simulink model "np"  (R2024a)
settings: Solver=VariableStepAuto  StartTime=0.0  StopTime=4000  RelTol=1e-3
libraries: aerolibatmos2 x25, simulink x1
(part 2 of 3)

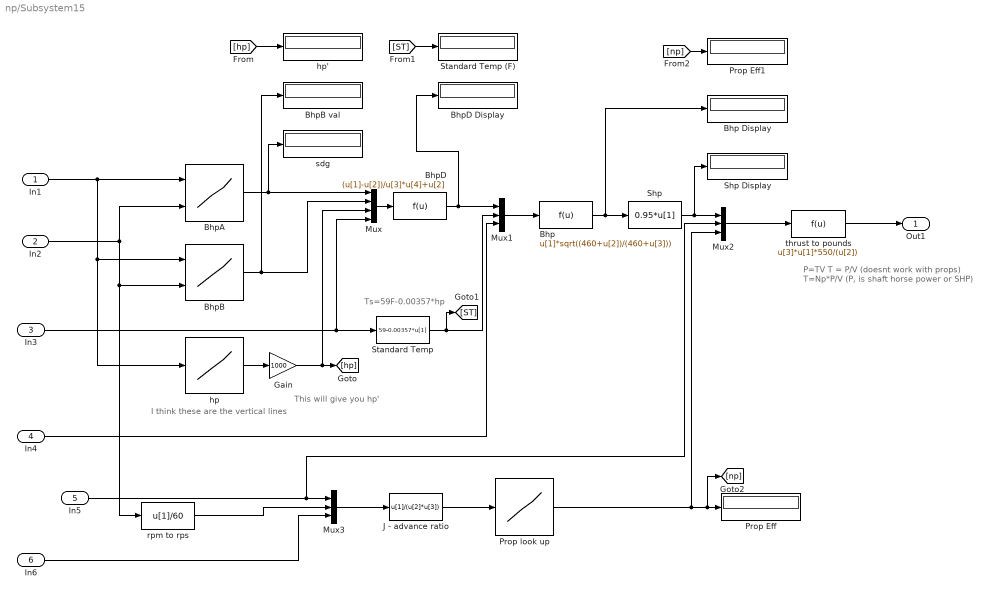
== system np/Subsystem15 ==
  note: This will give you hp'
  note: P=TV
      |
      | T = P/V (doesnt work with props)
      | T=Np*P/V (P, is shaft horse power or SHP)
  note: Ts=59F-0.00357*hp
  note: I think these are the vertical lines
  In1 : Inport
  In2 : Inport  Port=2
  In3 : Inport  Port=3
  In4 : Inport  Port=4
  In5 : Inport  Port=5
  In6 : Inport  Port=6
  Bhp : Fcn  Expr=u[1]*sqrt((460+u[2])/(460+u[3]))
  Bhp Display : Display
  BhpA : Lookup_n-D  BreakpointsForDimension1=[12;14;16;18;20;22;24;26;28]  BreakpointsForDimension2=[2000 2200 2400 2600 2700]  Table=[55 65 68 70 71;69 77 82 84 87;79 87 94 97 100;88 98 105 111 115;98 108 116 123 126;108 119 127 135 140;119 129 138 147 153;127 139 150 160 164;138 149 161 172 177]  InternalRulePriority=Speed  RndMeth=Simplest
      settings: InputPortMap=u0,u1
  BhpB : Lookup_n-D  BreakpointsForDimension1=[17 18 19 20 21 22 23 24 25 26 27 28 29]  BreakpointsForDimension2=[2000 2200 2400 2600 2700]  Table=[60 68 71 81 82;65 74 80 98 90;73 81 86 95 98;80 87 94 103 106;85 95 102 111 116;93 103 110 120 123;100 110 118 126 133;106 115 125 135 141;116 124 135 144 150;120 131 143 152 158;125 137 148 159 165;135 145 157 167 173;142 153 165 176 183]  InternalRulePriority=Speed  RndMeth=Simplest
      settings: InputPortMap=u0,u1
  BhpB val : Display
  BhpD : Fcn  Expr=(u[1]-u[2])/u[3]*u[4]+u[2]
  BhpD Display : Display
  Gain : Gain  Gain=1000
  J - advance ratio : Fcn  Expr=u[1]/(u[2]*u[3])
  Mux : Mux
  Mux1 : Mux  Inputs=3
  Mux2 : Mux  Inputs=3
  Mux3 : Mux  Inputs=3
  Prop Eff : Display
  Prop Eff1 : Display
  Prop look up : Lookup_n-D  NumberOfTableDimensions=1  BreakpointsForDimension1=[0;0.048012249;0.060807878;0.079983697;0.105563205;0.133281193;0.157430152;0.178753263;0.199368443;0.215001671;0.227800237;0.245557257;0.273971426;0.300949171;0.327207235;0.352754431;0.371192944;0.390339388;0.409494645;0.433608354;0.457002383;0.472603298;0.491041811;0.509471512;0.534281402;0.552003172;0.576810125;0.598782418;0.619332973;0.645549913;0.671763915;0.690895672;0.717103799;0.745432781;0.760302266;0.778708467;0.799946391;0.819051711;0.845926644;0.867848999;0.888343743;0.903180915;0.92013013;0.934250559;0.947645432;0.961736487;0.970184657;0.980736057;0.986337817;0.992650444;0.994753675]  Table=[0;0.109900628;0.134509301;0.163123953;0.206809061;0.257361734;0.294163365;0.333794761;0.373442069;0.400753217;0.42674495;0.454008364;0.499012887;0.534367813;0.564206411;0.592677861;0.607477825;0.622261878;0.641195111;0.661400024;0.676088609;0.688186099;0.702986063;0.713636848;0.72829361;0.738960306;0.752234009;0.764188297;0.773408288;0.783884048;0.792976749;0.800845502;0.807172083;0.81206787;0.813116793;0.812703099;0.812225759;0.807646975;0.794594806;0.783037077;0.765978931;0.751814195;0.732069486;0.713771482;0.68719103;0.655062427;0.632742534;0.600693488;0.571521941;0.543717542;0.53398839]  InternalRulePriority=Speed  RndMeth=Simplest
  Shp : Fcn  Expr=0.95*u[1]
  Shp Display : Display
  Standard Temp : Fcn  Expr=59-0.00357*u[1]
  Standard Temp (F) : Display
  hp : Lookup_n-D  NumberOfTableDimensions=1  BreakpointsForDimension1=[12, 14, 16, 18, 20, 22, 24, 26, 28]  Table=[22.5, 19.3, 15.8, 12.8, 10.3, 7.8, 5.5, 3.25, 1.4]  InternalRulePriority=Speed  RndMeth=Simplest
  "hp' " : Display
  rpm to rps : Fcn  Expr=u[1]/60
  sdg : Display
  thrust to pounds : Fcn  Expr=u[3]*u[1]*550/(u[2])
  Out1 : Outport
  wires:
  In6/1 -> Mux3/3
  In4/1 -> Mux1/3
  BhpA/1 -> Mux/1, sdg/1
  BhpD/1 -> Mux1/1, BhpD Display/1
  Mux2/1 -> thrust to pounds/1
  In5/1 -> Mux3/1, Mux2/2
  Bhp/1 -> Shp/1, Bhp Display/1
  thrust to pounds/1 -> Out1/1
  In3/1 -> Standard Temp/1, Mux/4
  Standard Temp/1 -> Mux1/2, [ST]
  BhpB/1 -> Mux/2, BhpB val/1
  Mux1/1 -> Bhp/1
  In2/1 -> rpm to rps/1, BhpB/2, BhpA/2
  In1/1 -> BhpA/1, BhpB/1, hp/1
  Shp/1 -> Mux2/1, Shp Display/1
  [np] -> Prop Eff1/1
  J - advance ratio/1 -> Prop look up/1
  Prop look up/1 -> Mux2/3, Prop Eff/1, [np]
  Mux/1 -> BhpD/1
  rpm to rps/1 -> Mux3/2
  [hp] -> "hp' "/1
  Mux3/1 -> J - advance ratio/1
  [ST] -> Standard Temp (F)/1
  Gain/1 -> Mux/3, [hp]
  hp/1 -> Gain/1

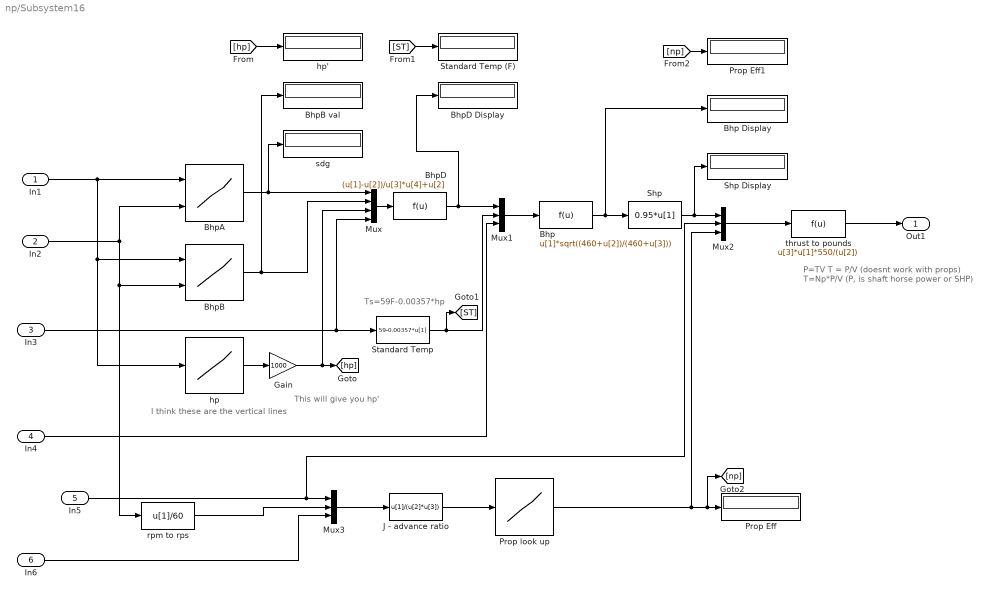
== system np/Subsystem16 ==
  note: This will give you hp'
  note: P=TV
      |
      | T = P/V (doesnt work with props)
      | T=Np*P/V (P, is shaft horse power or SHP)
  note: Ts=59F-0.00357*hp
  note: I think these are the vertical lines
  In1 : Inport
  In2 : Inport  Port=2
  In3 : Inport  Port=3
  In4 : Inport  Port=4
  In5 : Inport  Port=5
  In6 : Inport  Port=6
  Bhp : Fcn  Expr=u[1]*sqrt((460+u[2])/(460+u[3]))
  Bhp Display : Display
  BhpA : Lookup_n-D  BreakpointsForDimension1=[12;14;16;18;20;22;24;26;28]  BreakpointsForDimension2=[2000 2200 2400 2600 2700]  Table=[55 65 68 70 71;69 77 82 84 87;79 87 94 97 100;88 98 105 111 115;98 108 116 123 126;108 119 127 135 140;119 129 138 147 153;127 139 150 160 164;138 149 161 172 177]  InternalRulePriority=Speed  RndMeth=Simplest
      settings: InputPortMap=u0,u1
  BhpB : Lookup_n-D  BreakpointsForDimension1=[17 18 19 20 21 22 23 24 25 26 27 28 29]  BreakpointsForDimension2=[2000 2200 2400 2600 2700]  Table=[60 68 71 81 82;65 74 80 98 90;73 81 86 95 98;80 87 94 103 106;85 95 102 111 116;93 103 110 120 123;100 110 118 126 133;106 115 125 135 141;116 124 135 144 150;120 131 143 152 158;125 137 148 159 165;135 145 157 167 173;142 153 165 176 183]  InternalRulePriority=Speed  RndMeth=Simplest
      settings: InputPortMap=u0,u1
  BhpB val : Display
  BhpD : Fcn  Expr=(u[1]-u[2])/u[3]*u[4]+u[2]
  BhpD Display : Display
  Gain : Gain  Gain=1000
  J - advance ratio : Fcn  Expr=u[1]/(u[2]*u[3])
  Mux : Mux
  Mux1 : Mux  Inputs=3
  Mux2 : Mux  Inputs=3
  Mux3 : Mux  Inputs=3
  Prop Eff : Display
  Prop Eff1 : Display
  Prop look up : Lookup_n-D  NumberOfTableDimensions=1  BreakpointsForDimension1=[0;0.048012249;0.060807878;0.079983697;0.105563205;0.133281193;0.157430152;0.178753263;0.199368443;0.215001671;0.227800237;0.245557257;0.273971426;0.300949171;0.327207235;0.352754431;0.371192944;0.390339388;0.409494645;0.433608354;0.457002383;0.472603298;0.491041811;0.509471512;0.534281402;0.552003172;0.576810125;0.598782418;0.619332973;0.645549913;0.671763915;0.690895672;0.717103799;0.745432781;0.760302266;0.778708467;0.799946391;0.819051711;0.845926644;0.867848999;0.888343743;0.903180915;0.92013013;0.934250559;0.947645432;0.961736487;0.970184657;0.980736057;0.986337817;0.992650444;0.994753675]  Table=[0;0.109900628;0.134509301;0.163123953;0.206809061;0.257361734;0.294163365;0.333794761;0.373442069;0.400753217;0.42674495;0.454008364;0.499012887;0.534367813;0.564206411;0.592677861;0.607477825;0.622261878;0.641195111;0.661400024;0.676088609;0.688186099;0.702986063;0.713636848;0.72829361;0.738960306;0.752234009;0.764188297;0.773408288;0.783884048;0.792976749;0.800845502;0.807172083;0.81206787;0.813116793;0.812703099;0.812225759;0.807646975;0.794594806;0.783037077;0.765978931;0.751814195;0.732069486;0.713771482;0.68719103;0.655062427;0.632742534;0.600693488;0.571521941;0.543717542;0.53398839]  InternalRulePriority=Speed  RndMeth=Simplest
  Shp : Fcn  Expr=0.95*u[1]
  Shp Display : Display
  Standard Temp : Fcn  Expr=59-0.00357*u[1]
  Standard Temp (F) : Display
  hp : Lookup_n-D  NumberOfTableDimensions=1  BreakpointsForDimension1=[12, 14, 16, 18, 20, 22, 24, 26, 28]  Table=[22.5, 19.3, 15.8, 12.8, 10.3, 7.8, 5.5, 3.25, 1.4]  InternalRulePriority=Speed  RndMeth=Simplest
  "hp' " : Display
  rpm to rps : Fcn  Expr=u[1]/60
  sdg : Display
  thrust to pounds : Fcn  Expr=u[3]*u[1]*550/(u[2])
  Out1 : Outport
  wires:
  In6/1 -> Mux3/3
  In4/1 -> Mux1/3
  BhpA/1 -> Mux/1, sdg/1
  BhpD/1 -> Mux1/1, BhpD Display/1
  Mux2/1 -> thrust to pounds/1
  In5/1 -> Mux3/1, Mux2/2
  Bhp/1 -> Shp/1, Bhp Display/1
  thrust to pounds/1 -> Out1/1
  In3/1 -> Standard Temp/1, Mux/4
  Standard Temp/1 -> Mux1/2, [ST]
  BhpB/1 -> Mux/2, BhpB val/1
  Mux1/1 -> Bhp/1
  In2/1 -> rpm to rps/1, BhpB/2, BhpA/2
  In1/1 -> BhpA/1, BhpB/1, hp/1
  Shp/1 -> Mux2/1, Shp Display/1
  [np] -> Prop Eff1/1
  J - advance ratio/1 -> Prop look up/1
  Prop look up/1 -> Mux2/3, Prop Eff/1, [np]
  Mux/1 -> BhpD/1
  rpm to rps/1 -> Mux3/2
  [hp] -> "hp' "/1
  Mux3/1 -> J - advance ratio/1
  [ST] -> Standard Temp (F)/1
  Gain/1 -> Mux/3, [hp]
  hp/1 -> Gain/1

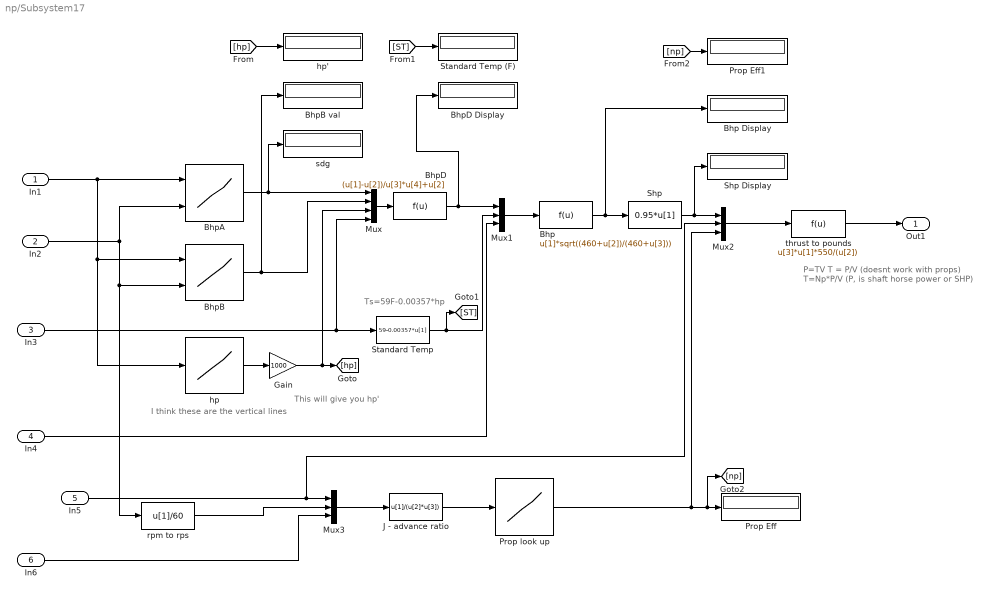
== system np/Subsystem17 ==
  note: I think these are the vertical lines
  note: Ts=59F-0.00357*hp
  note: P=TV
      |
      | T = P/V (doesnt work with props)
      | T=Np*P/V (P, is shaft horse power or SHP)
  note: This will give you hp'
  In1 : Inport
  In2 : Inport  Port=2
  In3 : Inport  Port=3
  In4 : Inport  Port=4
  In5 : Inport  Port=5
  In6 : Inport  Port=6
  Bhp : Fcn  Expr=u[1]*sqrt((460+u[2])/(460+u[3]))
  Bhp Display : Display
  BhpA : Lookup_n-D  BreakpointsForDimension1=[12;14;16;18;20;22;24;26;28]  BreakpointsForDimension2=[2000 2200 2400 2600 2700]  Table=[55 65 68 70 71;69 77 82 84 87;79 87 94 97 100;88 98 105 111 115;98 108 116 123 126;108 119 127 135 140;119 129 138 147 153;127 139 150 160 164;138 149 161 172 177]  InternalRulePriority=Speed  RndMeth=Simplest
      settings: InputPortMap=u0,u1
  BhpB : Lookup_n-D  BreakpointsForDimension1=[17 18 19 20 21 22 23 24 25 26 27 28 29]  BreakpointsForDimension2=[2000 2200 2400 2600 2700]  Table=[60 68 71 81 82;65 74 80 98 90;73 81 86 95 98;80 87 94 103 106;85 95 102 111 116;93 103 110 120 123;100 110 118 126 133;106 115 125 135 141;116 124 135 144 150;120 131 143 152 158;125 137 148 159 165;135 145 157 167 173;142 153 165 176 183]  InternalRulePriority=Speed  RndMeth=Simplest
      settings: InputPortMap=u0,u1
  BhpB val : Display
  BhpD : Fcn  Expr=(u[1]-u[2])/u[3]*u[4]+u[2]
  BhpD Display : Display
  Gain : Gain  Gain=1000
  J - advance ratio : Fcn  Expr=u[1]/(u[2]*u[3])
  Mux : Mux
  Mux1 : Mux  Inputs=3
  Mux2 : Mux  Inputs=3
  Mux3 : Mux  Inputs=3
  Prop Eff : Display
  Prop Eff1 : Display
  Prop look up : Lookup_n-D  NumberOfTableDimensions=1  BreakpointsForDimension1=[0;0.048012249;0.060807878;0.079983697;0.105563205;0.133281193;0.157430152;0.178753263;0.199368443;0.215001671;0.227800237;0.245557257;0.273971426;0.300949171;0.327207235;0.352754431;0.371192944;0.390339388;0.409494645;0.433608354;0.457002383;0.472603298;0.491041811;0.509471512;0.534281402;0.552003172;0.576810125;0.598782418;0.619332973;0.645549913;0.671763915;0.690895672;0.717103799;0.745432781;0.760302266;0.778708467;0.799946391;0.819051711;0.845926644;0.867848999;0.888343743;0.903180915;0.92013013;0.934250559;0.947645432;0.961736487;0.970184657;0.980736057;0.986337817;0.992650444;0.994753675]  Table=[0;0.109900628;0.134509301;0.163123953;0.206809061;0.257361734;0.294163365;0.333794761;0.373442069;0.400753217;0.42674495;0.454008364;0.499012887;0.534367813;0.564206411;0.592677861;0.607477825;0.622261878;0.641195111;0.661400024;0.676088609;0.688186099;0.702986063;0.713636848;0.72829361;0.738960306;0.752234009;0.764188297;0.773408288;0.783884048;0.792976749;0.800845502;0.807172083;0.81206787;0.813116793;0.812703099;0.812225759;0.807646975;0.794594806;0.783037077;0.765978931;0.751814195;0.732069486;0.713771482;0.68719103;0.655062427;0.632742534;0.600693488;0.571521941;0.543717542;0.53398839]  InternalRulePriority=Speed  RndMeth=Simplest
  Shp : Fcn  Expr=0.95*u[1]
  Shp Display : Display
  Standard Temp : Fcn  Expr=59-0.00357*u[1]
  Standard Temp (F) : Display
  hp : Lookup_n-D  NumberOfTableDimensions=1  BreakpointsForDimension1=[12, 14, 16, 18, 20, 22, 24, 26, 28]  Table=[22.5, 19.3, 15.8, 12.8, 10.3, 7.8, 5.5, 3.25, 1.4]  InternalRulePriority=Speed  RndMeth=Simplest
  "hp' " : Display
  rpm to rps : Fcn  Expr=u[1]/60
  sdg : Display
  thrust to pounds : Fcn  Expr=u[3]*u[1]*550/(u[2])
  Out1 : Outport
  wires:
  hp/1 -> Gain/1
  Gain/1 -> [hp], Mux/3
  [ST] -> Standard Temp (F)/1
  Mux3/1 -> J - advance ratio/1
  [hp] -> "hp' "/1
  rpm to rps/1 -> Mux3/2
  Mux/1 -> BhpD/1
  Prop look up/1 -> [np], Prop Eff/1, Mux2/3
  J - advance ratio/1 -> Prop look up/1
  [np] -> Prop Eff1/1
  Shp/1 -> Shp Display/1, Mux2/1
  In1/1 -> hp/1, BhpB/1, BhpA/1
  In2/1 -> BhpA/2, BhpB/2, rpm to rps/1
  Mux1/1 -> Bhp/1
  BhpB/1 -> BhpB val/1, Mux/2
  Standard Temp/1 -> [ST], Mux1/2
  In3/1 -> Mux/4, Standard Temp/1
  thrust to pounds/1 -> Out1/1
  Bhp/1 -> Bhp Display/1, Shp/1
  In5/1 -> Mux2/2, Mux3/1
  Mux2/1 -> thrust to pounds/1
  BhpD/1 -> BhpD Display/1, Mux1/1
  BhpA/1 -> sdg/1, Mux/1
  In4/1 -> Mux1/3
  In6/1 -> Mux3/3

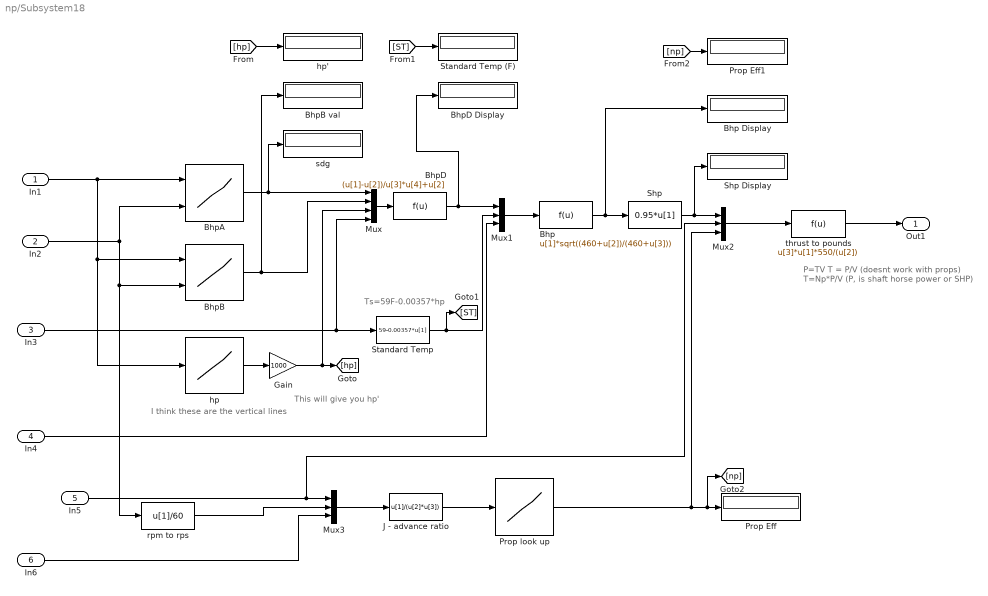
== system np/Subsystem18 ==
  note: This will give you hp'
  note: P=TV
      |
      | T = P/V (doesnt work with props)
      | T=Np*P/V (P, is shaft horse power or SHP)
  note: Ts=59F-0.00357*hp
  note: I think these are the vertical lines
  In1 : Inport
  In2 : Inport  Port=2
  In3 : Inport  Port=3
  In4 : Inport  Port=4
  In5 : Inport  Port=5
  In6 : Inport  Port=6
  Bhp : Fcn  Expr=u[1]*sqrt((460+u[2])/(460+u[3]))
  Bhp Display : Display
  BhpA : Lookup_n-D  BreakpointsForDimension1=[12;14;16;18;20;22;24;26;28]  BreakpointsForDimension2=[2000 2200 2400 2600 2700]  Table=[55 65 68 70 71;69 77 82 84 87;79 87 94 97 100;88 98 105 111 115;98 108 116 123 126;108 119 127 135 140;119 129 138 147 153;127 139 150 160 164;138 149 161 172 177]  InternalRulePriority=Speed  RndMeth=Simplest
      settings: InputPortMap=u0,u1
  BhpB : Lookup_n-D  BreakpointsForDimension1=[17 18 19 20 21 22 23 24 25 26 27 28 29]  BreakpointsForDimension2=[2000 2200 2400 2600 2700]  Table=[60 68 71 81 82;65 74 80 98 90;73 81 86 95 98;80 87 94 103 106;85 95 102 111 116;93 103 110 120 123;100 110 118 126 133;106 115 125 135 141;116 124 135 144 150;120 131 143 152 158;125 137 148 159 165;135 145 157 167 173;142 153 165 176 183]  InternalRulePriority=Speed  RndMeth=Simplest
      settings: InputPortMap=u0,u1
  BhpB val : Display
  BhpD : Fcn  Expr=(u[1]-u[2])/u[3]*u[4]+u[2]
  BhpD Display : Display
  Gain : Gain  Gain=1000
  J - advance ratio : Fcn  Expr=u[1]/(u[2]*u[3])
  Mux : Mux
  Mux1 : Mux  Inputs=3
  Mux2 : Mux  Inputs=3
  Mux3 : Mux  Inputs=3
  Prop Eff : Display
  Prop Eff1 : Display
  Prop look up : Lookup_n-D  NumberOfTableDimensions=1  BreakpointsForDimension1=[0;0.048012249;0.060807878;0.079983697;0.105563205;0.133281193;0.157430152;0.178753263;0.199368443;0.215001671;0.227800237;0.245557257;0.273971426;0.300949171;0.327207235;0.352754431;0.371192944;0.390339388;0.409494645;0.433608354;0.457002383;0.472603298;0.491041811;0.509471512;0.534281402;0.552003172;0.576810125;0.598782418;0.619332973;0.645549913;0.671763915;0.690895672;0.717103799;0.745432781;0.760302266;0.778708467;0.799946391;0.819051711;0.845926644;0.867848999;0.888343743;0.903180915;0.92013013;0.934250559;0.947645432;0.961736487;0.970184657;0.980736057;0.986337817;0.992650444;0.994753675]  Table=[0;0.109900628;0.134509301;0.163123953;0.206809061;0.257361734;0.294163365;0.333794761;0.373442069;0.400753217;0.42674495;0.454008364;0.499012887;0.534367813;0.564206411;0.592677861;0.607477825;0.622261878;0.641195111;0.661400024;0.676088609;0.688186099;0.702986063;0.713636848;0.72829361;0.738960306;0.752234009;0.764188297;0.773408288;0.783884048;0.792976749;0.800845502;0.807172083;0.81206787;0.813116793;0.812703099;0.812225759;0.807646975;0.794594806;0.783037077;0.765978931;0.751814195;0.732069486;0.713771482;0.68719103;0.655062427;0.632742534;0.600693488;0.571521941;0.543717542;0.53398839]  InternalRulePriority=Speed  RndMeth=Simplest
  Shp : Fcn  Expr=0.95*u[1]
  Shp Display : Display
  Standard Temp : Fcn  Expr=59-0.00357*u[1]
  Standard Temp (F) : Display
  hp : Lookup_n-D  NumberOfTableDimensions=1  BreakpointsForDimension1=[12, 14, 16, 18, 20, 22, 24, 26, 28]  Table=[22.5, 19.3, 15.8, 12.8, 10.3, 7.8, 5.5, 3.25, 1.4]  InternalRulePriority=Speed  RndMeth=Simplest
  "hp' " : Display
  rpm to rps : Fcn  Expr=u[1]/60
  sdg : Display
  thrust to pounds : Fcn  Expr=u[3]*u[1]*550/(u[2])
  Out1 : Outport
  wires:
  In6/1 -> Mux3/3
  In4/1 -> Mux1/3
  BhpA/1 -> Mux/1, sdg/1
  BhpD/1 -> Mux1/1, BhpD Display/1
  Mux2/1 -> thrust to pounds/1
  In5/1 -> Mux3/1, Mux2/2
  Bhp/1 -> Shp/1, Bhp Display/1
  thrust to pounds/1 -> Out1/1
  In3/1 -> Standard Temp/1, Mux/4
  Standard Temp/1 -> Mux1/2, [ST]
  BhpB/1 -> Mux/2, BhpB val/1
  Mux1/1 -> Bhp/1
  In2/1 -> rpm to rps/1, BhpB/2, BhpA/2
  In1/1 -> BhpA/1, BhpB/1, hp/1
  Shp/1 -> Mux2/1, Shp Display/1
  [np] -> Prop Eff1/1
  J - advance ratio/1 -> Prop look up/1
  Prop look up/1 -> Mux2/3, Prop Eff/1, [np]
  Mux/1 -> BhpD/1
  rpm to rps/1 -> Mux3/2
  [hp] -> "hp' "/1
  Mux3/1 -> J - advance ratio/1
  [ST] -> Standard Temp (F)/1
  Gain/1 -> Mux/3, [hp]
  hp/1 -> Gain/1

== system np/Subsystem19 ==
  note: This will give you hp'
  note: P=TV
      |
      | T = P/V (doesnt work with props)
      | T=Np*P/V (P, is shaft horse power or SHP)
  note: Ts=59F-0.00357*hp
  note: I think these are the vertical lines
  In1 : Inport
  In2 : Inport  Port=2
  In3 : Inport  Port=3
  In4 : Inport  Port=4
  In5 : Inport  Port=5
  In6 : Inport  Port=6
  Bhp : Fcn  Expr=u[1]*sqrt((460+u[2])/(460+u[3]))
  Bhp Display : Display
  BhpA : Lookup_n-D  BreakpointsForDimension1=[12;14;16;18;20;22;24;26;28]  BreakpointsForDimension2=[2000 2200 2400 2600 2700]  Table=[55 65 68 70 71;69 77 82 84 87;79 87 94 97 100;88 98 105 111 115;98 108 116 123 126;108 119 127 135 140;119 129 138 147 153;127 139 150 160 164;138 149 161 172 177]  InternalRulePriority=Speed  RndMeth=Simplest
      settings: InputPortMap=u0,u1
  BhpB : Lookup_n-D  BreakpointsForDimension1=[17 18 19 20 21 22 23 24 25 26 27 28 29]  BreakpointsForDimension2=[2000 2200 2400 2600 2700]  Table=[60 68 71 81 82;65 74 80 98 90;73 81 86 95 98;80 87 94 103 106;85 95 102 111 116;93 103 110 120 123;100 110 118 126 133;106 115 125 135 141;116 124 135 144 150;120 131 143 152 158;125 137 148 159 165;135 145 157 167 173;142 153 165 176 183]  InternalRulePriority=Speed  RndMeth=Simplest
      settings: InputPortMap=u0,u1
  BhpB val : Display
  BhpD : Fcn  Expr=(u[1]-u[2])/u[3]*u[4]+u[2]
  BhpD Display : Display
  Gain : Gain  Gain=1000
  J - advance ratio : Fcn  Expr=u[1]/(u[2]*u[3])
  Mux : Mux
  Mux1 : Mux  Inputs=3
  Mux2 : Mux  Inputs=3
  Mux3 : Mux  Inputs=3
  Prop Eff : Display
  Prop Eff1 : Display
  Prop look up : Lookup_n-D  NumberOfTableDimensions=1  BreakpointsForDimension1=[0;0.048012249;0.060807878;0.079983697;0.105563205;0.133281193;0.157430152;0.178753263;0.199368443;0.215001671;0.227800237;0.245557257;0.273971426;0.300949171;0.327207235;0.352754431;0.371192944;0.390339388;0.409494645;0.433608354;0.457002383;0.472603298;0.491041811;0.509471512;0.534281402;0.552003172;0.576810125;0.598782418;0.619332973;0.645549913;0.671763915;0.690895672;0.717103799;0.745432781;0.760302266;0.778708467;0.799946391;0.819051711;0.845926644;0.867848999;0.888343743;0.903180915;0.92013013;0.934250559;0.947645432;0.961736487;0.970184657;0.980736057;0.986337817;0.992650444;0.994753675]  Table=[0;0.109900628;0.134509301;0.163123953;0.206809061;0.257361734;0.294163365;0.333794761;0.373442069;0.400753217;0.42674495;0.454008364;0.499012887;0.534367813;0.564206411;0.592677861;0.607477825;0.622261878;0.641195111;0.661400024;0.676088609;0.688186099;0.702986063;0.713636848;0.72829361;0.738960306;0.752234009;0.764188297;0.773408288;0.783884048;0.792976749;0.800845502;0.807172083;0.81206787;0.813116793;0.812703099;0.812225759;0.807646975;0.794594806;0.783037077;0.765978931;0.751814195;0.732069486;0.713771482;0.68719103;0.655062427;0.632742534;0.600693488;0.571521941;0.543717542;0.53398839]  InternalRulePriority=Speed  RndMeth=Simplest
  Shp : Fcn  Expr=0.95*u[1]
  Shp Display : Display
  Standard Temp : Fcn  Expr=59-0.00357*u[1]
  Standard Temp (F) : Display
  hp : Lookup_n-D  NumberOfTableDimensions=1  BreakpointsForDimension1=[12, 14, 16, 18, 20, 22, 24, 26, 28]  Table=[22.5, 19.3, 15.8, 12.8, 10.3, 7.8, 5.5, 3.25, 1.4]  InternalRulePriority=Speed  RndMeth=Simplest
  "hp' " : Display
  rpm to rps : Fcn  Expr=u[1]/60
  sdg : Display
  thrust to pounds : Fcn  Expr=u[3]*u[1]*550/(u[2])
  Out1 : Outport
  wires:
  In6/1 -> Mux3/3
  In4/1 -> Mux1/3
  BhpA/1 -> Mux/1, sdg/1
  BhpD/1 -> Mux1/1, BhpD Display/1
  Mux2/1 -> thrust to pounds/1
  In5/1 -> Mux3/1, Mux2/2
  Bhp/1 -> Shp/1, Bhp Display/1
  thrust to pounds/1 -> Out1/1
  In3/1 -> Standard Temp/1, Mux/4
  Standard Temp/1 -> Mux1/2, [ST]
  BhpB/1 -> Mux/2, BhpB val/1
  Mux1/1 -> Bhp/1
  In2/1 -> rpm to rps/1, BhpB/2, BhpA/2
  In1/1 -> BhpA/1, BhpB/1, hp/1
  Shp/1 -> Mux2/1, Shp Display/1
  [np] -> Prop Eff1/1
  J - advance ratio/1 -> Prop look up/1
  Prop look up/1 -> Mux2/3, Prop Eff/1, [np]
  Mux/1 -> BhpD/1
  rpm to rps/1 -> Mux3/2
  [hp] -> "hp' "/1
  Mux3/1 -> J - advance ratio/1
  [ST] -> Standard Temp (F)/1
  Gain/1 -> Mux/3, [hp]
  hp/1 -> Gain/1

== system np/Subsystem2 ==
  note: This will give you hp'
  note: P=TV
      |
      | T = P/V (doesnt work with props)
      | T=Np*P/V (P, is shaft horse power or SHP)
  note: Ts=59F-0.00357*hp
  note: I think these are the vertical lines
  In1 : Inport
  In2 : Inport  Port=2
  In3 : Inport  Port=3
  In4 : Inport  Port=4
  In5 : Inport  Port=5
  In6 : Inport  Port=6
  Bhp : Fcn  Expr=u[1]*sqrt((460+u[2])/(460+u[3]))
  Bhp Display : Display
  BhpA : Lookup_n-D  BreakpointsForDimension1=[12;14;16;18;20;22;24;26;28]  BreakpointsForDimension2=[2000 2200 2400 2600 2700]  Table=[55 65 68 70 71;69 77 82 84 87;79 87 94 97 100;88 98 105 111 115;98 108 116 123 126;108 119 127 135 140;119 129 138 147 153;127 139 150 160 164;138 149 161 172 177]  InternalRulePriority=Speed  RndMeth=Simplest
      settings: InputPortMap=u0,u1
  BhpB : Lookup_n-D  BreakpointsForDimension1=[17 18 19 20 21 22 23 24 25 26 27 28 29]  BreakpointsForDimension2=[2000 2200 2400 2600 2700]  Table=[60 68 71 81 82;65 74 80 98 90;73 81 86 95 98;80 87 94 103 106;85 95 102 111 116;93 103 110 120 123;100 110 118 126 133;106 115 125 135 141;116 124 135 144 150;120 131 143 152 158;125 137 148 159 165;135 145 157 167 173;142 153 165 176 183]  InternalRulePriority=Speed  RndMeth=Simplest
      settings: InputPortMap=u0,u1
  BhpB val : Display
  BhpD : Fcn  Expr=(u[1]-u[2])/u[3]*u[4]+u[2]
  BhpD Display : Display
  Gain : Gain  Gain=1000
  J - advance ratio : Fcn  Expr=u[1]/(u[2]*u[3])
  Mux : Mux
  Mux1 : Mux  Inputs=3
  Mux2 : Mux  Inputs=3
  Mux3 : Mux  Inputs=3
  Prop Eff : Display
  Prop Eff1 : Display
  Prop look up : Lookup_n-D  NumberOfTableDimensions=1  BreakpointsForDimension1=[0;0.048012249;0.060807878;0.079983697;0.105563205;0.133281193;0.157430152;0.178753263;0.199368443;0.215001671;0.227800237;0.245557257;0.273971426;0.300949171;0.327207235;0.352754431;0.371192944;0.390339388;0.409494645;0.433608354;0.457002383;0.472603298;0.491041811;0.509471512;0.534281402;0.552003172;0.576810125;0.598782418;0.619332973;0.645549913;0.671763915;0.690895672;0.717103799;0.745432781;0.760302266;0.778708467;0.799946391;0.819051711;0.845926644;0.867848999;0.888343743;0.903180915;0.92013013;0.934250559;0.947645432;0.961736487;0.970184657;0.980736057;0.986337817;0.992650444;0.994753675]  Table=[0;0.109900628;0.134509301;0.163123953;0.206809061;0.257361734;0.294163365;0.333794761;0.373442069;0.400753217;0.42674495;0.454008364;0.499012887;0.534367813;0.564206411;0.592677861;0.607477825;0.622261878;0.641195111;0.661400024;0.676088609;0.688186099;0.702986063;0.713636848;0.72829361;0.738960306;0.752234009;0.764188297;0.773408288;0.783884048;0.792976749;0.800845502;0.807172083;0.81206787;0.813116793;0.812703099;0.812225759;0.807646975;0.794594806;0.783037077;0.765978931;0.751814195;0.732069486;0.713771482;0.68719103;0.655062427;0.632742534;0.600693488;0.571521941;0.543717542;0.53398839]  InternalRulePriority=Speed  RndMeth=Simplest
  Shp : Fcn  Expr=0.95*u[1]
  Shp Display : Display
  Standard Temp : Fcn  Expr=59-0.00357*u[1]
  Standard Temp (F) : Display
  hp : Lookup_n-D  NumberOfTableDimensions=1  BreakpointsForDimension1=[12, 14, 16, 18, 20, 22, 24, 26, 28]  Table=[22.5, 19.3, 15.8, 12.8, 10.3, 7.8, 5.5, 3.25, 1.4]  InternalRulePriority=Speed  RndMeth=Simplest
  "hp' " : Display
  rpm to rps : Fcn  Expr=u[1]/60
  sdg : Display
  thrust to pounds : Fcn  Expr=u[3]*u[1]*550/(u[2])
  Out1 : Outport
  wires:
  In6/1 -> Mux3/3
  In4/1 -> Mux1/3
  BhpA/1 -> Mux/1, sdg/1
  BhpD/1 -> Mux1/1, BhpD Display/1
  Mux2/1 -> thrust to pounds/1
  In5/1 -> Mux3/1, Mux2/2
  Bhp/1 -> Shp/1, Bhp Display/1
  thrust to pounds/1 -> Out1/1
  In3/1 -> Standard Temp/1, Mux/4
  Standard Temp/1 -> Mux1/2, [ST]
  BhpB/1 -> Mux/2, BhpB val/1
  Mux1/1 -> Bhp/1
  In2/1 -> rpm to rps/1, BhpB/2, BhpA/2
  In1/1 -> BhpA/1, BhpB/1, hp/1
  Shp/1 -> Mux2/1, Shp Display/1
  [np] -> Prop Eff1/1
  J - advance ratio/1 -> Prop look up/1
  Prop look up/1 -> Mux2/3, Prop Eff/1, [np]
  Mux/1 -> BhpD/1
  rpm to rps/1 -> Mux3/2
  [hp] -> "hp' "/1
  Mux3/1 -> J - advance ratio/1
  [ST] -> Standard Temp (F)/1
  Gain/1 -> Mux/3, [hp]
  hp/1 -> Gain/1

== system np/Subsystem20 ==
  note: This will give you hp'
  note: P=TV
      |
      | T = P/V (doesnt work with props)
      | T=Np*P/V (P, is shaft horse power or SHP)
  note: Ts=59F-0.00357*hp
  note: I think these are the vertical lines
  In1 : Inport
  In2 : Inport  Port=2
  In3 : Inport  Port=3
  In4 : Inport  Port=4
  In5 : Inport  Port=5
  In6 : Inport  Port=6
  Bhp : Fcn  Expr=u[1]*sqrt((460+u[2])/(460+u[3]))
  Bhp Display : Display
  BhpA : Lookup_n-D  BreakpointsForDimension1=[12;14;16;18;20;22;24;26;28]  BreakpointsForDimension2=[2000 2200 2400 2600 2700]  Table=[55 65 68 70 71;69 77 82 84 87;79 87 94 97 100;88 98 105 111 115;98 108 116 123 126;108 119 127 135 140;119 129 138 147 153;127 139 150 160 164;138 149 161 172 177]  InternalRulePriority=Speed  RndMeth=Simplest
      settings: InputPortMap=u0,u1
  BhpB : Lookup_n-D  BreakpointsForDimension1=[17 18 19 20 21 22 23 24 25 26 27 28 29]  BreakpointsForDimension2=[2000 2200 2400 2600 2700]  Table=[60 68 71 81 82;65 74 80 98 90;73 81 86 95 98;80 87 94 103 106;85 95 102 111 116;93 103 110 120 123;100 110 118 126 133;106 115 125 135 141;116 124 135 144 150;120 131 143 152 158;125 137 148 159 165;135 145 157 167 173;142 153 165 176 183]  InternalRulePriority=Speed  RndMeth=Simplest
      settings: InputPortMap=u0,u1
  BhpB val : Display
  BhpD : Fcn  Expr=(u[1]-u[2])/u[3]*u[4]+u[2]
  BhpD Display : Display
  Gain : Gain  Gain=1000
  J - advance ratio : Fcn  Expr=u[1]/(u[2]*u[3])
  Mux : Mux
  Mux1 : Mux  Inputs=3
  Mux2 : Mux  Inputs=3
  Mux3 : Mux  Inputs=3
  Prop Eff : Display
  Prop Eff1 : Display
  Prop look up : Lookup_n-D  NumberOfTableDimensions=1  BreakpointsForDimension1=[0;0.048012249;0.060807878;0.079983697;0.105563205;0.133281193;0.157430152;0.178753263;0.199368443;0.215001671;0.227800237;0.245557257;0.273971426;0.300949171;0.327207235;0.352754431;0.371192944;0.390339388;0.409494645;0.433608354;0.457002383;0.472603298;0.491041811;0.509471512;0.534281402;0.552003172;0.576810125;0.598782418;0.619332973;0.645549913;0.671763915;0.690895672;0.717103799;0.745432781;0.760302266;0.778708467;0.799946391;0.819051711;0.845926644;0.867848999;0.888343743;0.903180915;0.92013013;0.934250559;0.947645432;0.961736487;0.970184657;0.980736057;0.986337817;0.992650444;0.994753675]  Table=[0;0.109900628;0.134509301;0.163123953;0.206809061;0.257361734;0.294163365;0.333794761;0.373442069;0.400753217;0.42674495;0.454008364;0.499012887;0.534367813;0.564206411;0.592677861;0.607477825;0.622261878;0.641195111;0.661400024;0.676088609;0.688186099;0.702986063;0.713636848;0.72829361;0.738960306;0.752234009;0.764188297;0.773408288;0.783884048;0.792976749;0.800845502;0.807172083;0.81206787;0.813116793;0.812703099;0.812225759;0.807646975;0.794594806;0.783037077;0.765978931;0.751814195;0.732069486;0.713771482;0.68719103;0.655062427;0.632742534;0.600693488;0.571521941;0.543717542;0.53398839]  InternalRulePriority=Speed  RndMeth=Simplest
  Shp : Fcn  Expr=0.95*u[1]
  Shp Display : Display
  Standard Temp : Fcn  Expr=59-0.00357*u[1]
  Standard Temp (F) : Display
  hp : Lookup_n-D  NumberOfTableDimensions=1  BreakpointsForDimension1=[12, 14, 16, 18, 20, 22, 24, 26, 28]  Table=[22.5, 19.3, 15.8, 12.8, 10.3, 7.8, 5.5, 3.25, 1.4]  InternalRulePriority=Speed  RndMeth=Simplest
  "hp' " : Display
  rpm to rps : Fcn  Expr=u[1]/60
  sdg : Display
  thrust to pounds : Fcn  Expr=u[3]*u[1]*550/(u[2])
  Out1 : Outport
  wires:
  In6/1 -> Mux3/3
  In4/1 -> Mux1/3
  BhpA/1 -> Mux/1, sdg/1
  BhpD/1 -> Mux1/1, BhpD Display/1
  Mux2/1 -> thrust to pounds/1
  In5/1 -> Mux3/1, Mux2/2
  Bhp/1 -> Shp/1, Bhp Display/1
  thrust to pounds/1 -> Out1/1
  In3/1 -> Standard Temp/1, Mux/4
  Standard Temp/1 -> Mux1/2, [ST]
  BhpB/1 -> Mux/2, BhpB val/1
  Mux1/1 -> Bhp/1
  In2/1 -> rpm to rps/1, BhpB/2, BhpA/2
  In1/1 -> BhpA/1, BhpB/1, hp/1
  Shp/1 -> Mux2/1, Shp Display/1
  [np] -> Prop Eff1/1
  J - advance ratio/1 -> Prop look up/1
  Prop look up/1 -> Mux2/3, Prop Eff/1, [np]
  Mux/1 -> BhpD/1
  rpm to rps/1 -> Mux3/2
  [hp] -> "hp' "/1
  Mux3/1 -> J - advance ratio/1
  [ST] -> Standard Temp (F)/1
  Gain/1 -> Mux/3, [hp]
  hp/1 -> Gain/1

== system np/Subsystem21 ==
  note: I think these are the vertical lines
  note: Ts=59F-0.00357*hp
  note: P=TV
      |
      | T = P/V (doesnt work with props)
      | T=Np*P/V (P, is shaft horse power or SHP)
  note: This will give you hp'
  In1 : Inport
  In2 : Inport  Port=2
  In3 : Inport  Port=3
  In4 : Inport  Port=4
  In5 : Inport  Port=5
  In6 : Inport  Port=6
  Bhp : Fcn  Expr=u[1]*sqrt((460+u[2])/(460+u[3]))
  Bhp Display : Display
  BhpA : Lookup_n-D  BreakpointsForDimension1=[12;14;16;18;20;22;24;26;28]  BreakpointsForDimension2=[2000 2200 2400 2600 2700]  Table=[55 65 68 70 71;69 77 82 84 87;79 87 94 97 100;88 98 105 111 115;98 108 116 123 126;108 119 127 135 140;119 129 138 147 153;127 139 150 160 164;138 149 161 172 177]  InternalRulePriority=Speed  RndMeth=Simplest
      settings: InputPortMap=u0,u1
  BhpB : Lookup_n-D  BreakpointsForDimension1=[17 18 19 20 21 22 23 24 25 26 27 28 29]  BreakpointsForDimension2=[2000 2200 2400 2600 2700]  Table=[60 68 71 81 82;65 74 80 98 90;73 81 86 95 98;80 87 94 103 106;85 95 102 111 116;93 103 110 120 123;100 110 118 126 133;106 115 125 135 141;116 124 135 144 150;120 131 143 152 158;125 137 148 159 165;135 145 157 167 173;142 153 165 176 183]  InternalRulePriority=Speed  RndMeth=Simplest
      settings: InputPortMap=u0,u1
  BhpB val : Display
  BhpD : Fcn  Expr=(u[1]-u[2])/u[3]*u[4]+u[2]
  BhpD Display : Display
  Gain : Gain  Gain=1000
  J - advance ratio : Fcn  Expr=u[1]/(u[2]*u[3])
  Mux : Mux
  Mux1 : Mux  Inputs=3
  Mux2 : Mux  Inputs=3
  Mux3 : Mux  Inputs=3
  Prop Eff : Display
  Prop Eff1 : Display
  Prop look up : Lookup_n-D  NumberOfTableDimensions=1  BreakpointsForDimension1=[0;0.048012249;0.060807878;0.079983697;0.105563205;0.133281193;0.157430152;0.178753263;0.199368443;0.215001671;0.227800237;0.245557257;0.273971426;0.300949171;0.327207235;0.352754431;0.371192944;0.390339388;0.409494645;0.433608354;0.457002383;0.472603298;0.491041811;0.509471512;0.534281402;0.552003172;0.576810125;0.598782418;0.619332973;0.645549913;0.671763915;0.690895672;0.717103799;0.745432781;0.760302266;0.778708467;0.799946391;0.819051711;0.845926644;0.867848999;0.888343743;0.903180915;0.92013013;0.934250559;0.947645432;0.961736487;0.970184657;0.980736057;0.986337817;0.992650444;0.994753675]  Table=[0;0.109900628;0.134509301;0.163123953;0.206809061;0.257361734;0.294163365;0.333794761;0.373442069;0.400753217;0.42674495;0.454008364;0.499012887;0.534367813;0.564206411;0.592677861;0.607477825;0.622261878;0.641195111;0.661400024;0.676088609;0.688186099;0.702986063;0.713636848;0.72829361;0.738960306;0.752234009;0.764188297;0.773408288;0.783884048;0.792976749;0.800845502;0.807172083;0.81206787;0.813116793;0.812703099;0.812225759;0.807646975;0.794594806;0.783037077;0.765978931;0.751814195;0.732069486;0.713771482;0.68719103;0.655062427;0.632742534;0.600693488;0.571521941;0.543717542;0.53398839]  InternalRulePriority=Speed  RndMeth=Simplest
  Shp : Fcn  Expr=0.95*u[1]
  Shp Display : Display
  Standard Temp : Fcn  Expr=59-0.00357*u[1]
  Standard Temp (F) : Display
  hp : Lookup_n-D  NumberOfTableDimensions=1  BreakpointsForDimension1=[12, 14, 16, 18, 20, 22, 24, 26, 28]  Table=[22.5, 19.3, 15.8, 12.8, 10.3, 7.8, 5.5, 3.25, 1.4]  InternalRulePriority=Speed  RndMeth=Simplest
  "hp' " : Display
  rpm to rps : Fcn  Expr=u[1]/60
  sdg : Display
  thrust to pounds : Fcn  Expr=u[3]*u[1]*550/(u[2])
  Out1 : Outport
  wires:
  hp/1 -> Gain/1
  Gain/1 -> [hp], Mux/3
  [ST] -> Standard Temp (F)/1
  Mux3/1 -> J - advance ratio/1
  [hp] -> "hp' "/1
  rpm to rps/1 -> Mux3/2
  Mux/1 -> BhpD/1
  Prop look up/1 -> [np], Prop Eff/1, Mux2/3
  J - advance ratio/1 -> Prop look up/1
  [np] -> Prop Eff1/1
  Shp/1 -> Shp Display/1, Mux2/1
  In1/1 -> hp/1, BhpB/1, BhpA/1
  In2/1 -> BhpA/2, BhpB/2, rpm to rps/1
  Mux1/1 -> Bhp/1
  BhpB/1 -> BhpB val/1, Mux/2
  Standard Temp/1 -> [ST], Mux1/2
  In3/1 -> Mux/4, Standard Temp/1
  thrust to pounds/1 -> Out1/1
  Bhp/1 -> Bhp Display/1, Shp/1
  In5/1 -> Mux2/2, Mux3/1
  Mux2/1 -> thrust to pounds/1
  BhpD/1 -> BhpD Display/1, Mux1/1
  BhpA/1 -> sdg/1, Mux/1
  In4/1 -> Mux1/3
  In6/1 -> Mux3/3

== system np/Subsystem22 ==
  note: This will give you hp'
  note: P=TV
      |
      | T = P/V (doesnt work with props)
      | T=Np*P/V (P, is shaft horse power or SHP)
  note: Ts=59F-0.00357*hp
  note: I think these are the vertical lines
  In1 : Inport
  In2 : Inport  Port=2
  In3 : Inport  Port=3
  In4 : Inport  Port=4
  In5 : Inport  Port=5
  In6 : Inport  Port=6
  Bhp : Fcn  Expr=u[1]*sqrt((460+u[2])/(460+u[3]))
  Bhp Display : Display
  BhpA : Lookup_n-D  BreakpointsForDimension1=[12;14;16;18;20;22;24;26;28]  BreakpointsForDimension2=[2000 2200 2400 2600 2700]  Table=[55 65 68 70 71;69 77 82 84 87;79 87 94 97 100;88 98 105 111 115;98 108 116 123 126;108 119 127 135 140;119 129 138 147 153;127 139 150 160 164;138 149 161 172 177]  InternalRulePriority=Speed  RndMeth=Simplest
      settings: InputPortMap=u0,u1
  BhpB : Lookup_n-D  BreakpointsForDimension1=[17 18 19 20 21 22 23 24 25 26 27 28 29]  BreakpointsForDimension2=[2000 2200 2400 2600 2700]  Table=[60 68 71 81 82;65 74 80 98 90;73 81 86 95 98;80 87 94 103 106;85 95 102 111 116;93 103 110 120 123;100 110 118 126 133;106 115 125 135 141;116 124 135 144 150;120 131 143 152 158;125 137 148 159 165;135 145 157 167 173;142 153 165 176 183]  InternalRulePriority=Speed  RndMeth=Simplest
      settings: InputPortMap=u0,u1
  BhpB val : Display
  BhpD : Fcn  Expr=(u[1]-u[2])/u[3]*u[4]+u[2]
  BhpD Display : Display
  Gain : Gain  Gain=1000
  J - advance ratio : Fcn  Expr=u[1]/(u[2]*u[3])
  Mux : Mux
  Mux1 : Mux  Inputs=3
  Mux2 : Mux  Inputs=3
  Mux3 : Mux  Inputs=3
  Prop Eff : Display
  Prop Eff1 : Display
  Prop look up : Lookup_n-D  NumberOfTableDimensions=1  BreakpointsForDimension1=[0;0.048012249;0.060807878;0.079983697;0.105563205;0.133281193;0.157430152;0.178753263;0.199368443;0.215001671;0.227800237;0.245557257;0.273971426;0.300949171;0.327207235;0.352754431;0.371192944;0.390339388;0.409494645;0.433608354;0.457002383;0.472603298;0.491041811;0.509471512;0.534281402;0.552003172;0.576810125;0.598782418;0.619332973;0.645549913;0.671763915;0.690895672;0.717103799;0.745432781;0.760302266;0.778708467;0.799946391;0.819051711;0.845926644;0.867848999;0.888343743;0.903180915;0.92013013;0.934250559;0.947645432;0.961736487;0.970184657;0.980736057;0.986337817;0.992650444;0.994753675]  Table=[0;0.109900628;0.134509301;0.163123953;0.206809061;0.257361734;0.294163365;0.333794761;0.373442069;0.400753217;0.42674495;0.454008364;0.499012887;0.534367813;0.564206411;0.592677861;0.607477825;0.622261878;0.641195111;0.661400024;0.676088609;0.688186099;0.702986063;0.713636848;0.72829361;0.738960306;0.752234009;0.764188297;0.773408288;0.783884048;0.792976749;0.800845502;0.807172083;0.81206787;0.813116793;0.812703099;0.812225759;0.807646975;0.794594806;0.783037077;0.765978931;0.751814195;0.732069486;0.713771482;0.68719103;0.655062427;0.632742534;0.600693488;0.571521941;0.543717542;0.53398839]  InternalRulePriority=Speed  RndMeth=Simplest
  Shp : Fcn  Expr=0.95*u[1]
  Shp Display : Display
  Standard Temp : Fcn  Expr=59-0.00357*u[1]
  Standard Temp (F) : Display
  hp : Lookup_n-D  NumberOfTableDimensions=1  BreakpointsForDimension1=[12, 14, 16, 18, 20, 22, 24, 26, 28]  Table=[22.5, 19.3, 15.8, 12.8, 10.3, 7.8, 5.5, 3.25, 1.4]  InternalRulePriority=Speed  RndMeth=Simplest
  "hp' " : Display
  rpm to rps : Fcn  Expr=u[1]/60
  sdg : Display
  thrust to pounds : Fcn  Expr=u[3]*u[1]*550/(u[2])
  Out1 : Outport
  wires:
  In6/1 -> Mux3/3
  In4/1 -> Mux1/3
  BhpA/1 -> Mux/1, sdg/1
  BhpD/1 -> Mux1/1, BhpD Display/1
  Mux2/1 -> thrust to pounds/1
  In5/1 -> Mux3/1, Mux2/2
  Bhp/1 -> Shp/1, Bhp Display/1
  thrust to pounds/1 -> Out1/1
  In3/1 -> Standard Temp/1, Mux/4
  Standard Temp/1 -> Mux1/2, [ST]
  BhpB/1 -> Mux/2, BhpB val/1
  Mux1/1 -> Bhp/1
  In2/1 -> rpm to rps/1, BhpB/2, BhpA/2
  In1/1 -> BhpA/1, BhpB/1, hp/1
  Shp/1 -> Mux2/1, Shp Display/1
  [np] -> Prop Eff1/1
  J - advance ratio/1 -> Prop look up/1
  Prop look up/1 -> Mux2/3, Prop Eff/1, [np]
  Mux/1 -> BhpD/1
  rpm to rps/1 -> Mux3/2
  [hp] -> "hp' "/1
  Mux3/1 -> J - advance ratio/1
  [ST] -> Standard Temp (F)/1
  Gain/1 -> Mux/3, [hp]
  hp/1 -> Gain/1

== system np/Subsystem23 ==
  note: I think these are the vertical lines
  note: Ts=59F-0.00357*hp
  note: P=TV
      |
      | T = P/V (doesnt work with props)
      | T=Np*P/V (P, is shaft horse power or SHP)
  note: This will give you hp'
  In1 : Inport
  In2 : Inport  Port=2
  In3 : Inport  Port=3
  In4 : Inport  Port=4
  In5 : Inport  Port=5
  In6 : Inport  Port=6
  Bhp : Fcn  Expr=u[1]*sqrt((460+u[2])/(460+u[3]))
  Bhp Display : Display
  BhpA : Lookup_n-D  BreakpointsForDimension1=[12;14;16;18;20;22;24;26;28]  BreakpointsForDimension2=[2000 2200 2400 2600 2700]  Table=[55 65 68 70 71;69 77 82 84 87;79 87 94 97 100;88 98 105 111 115;98 108 116 123 126;108 119 127 135 140;119 129 138 147 153;127 139 150 160 164;138 149 161 172 177]  InternalRulePriority=Speed  RndMeth=Simplest
      settings: InputPortMap=u0,u1
  BhpB : Lookup_n-D  BreakpointsForDimension1=[17 18 19 20 21 22 23 24 25 26 27 28 29]  BreakpointsForDimension2=[2000 2200 2400 2600 2700]  Table=[60 68 71 81 82;65 74 80 98 90;73 81 86 95 98;80 87 94 103 106;85 95 102 111 116;93 103 110 120 123;100 110 118 126 133;106 115 125 135 141;116 124 135 144 150;120 131 143 152 158;125 137 148 159 165;135 145 157 167 173;142 153 165 176 183]  InternalRulePriority=Speed  RndMeth=Simplest
      settings: InputPortMap=u0,u1
  BhpB val : Display
  BhpD : Fcn  Expr=(u[1]-u[2])/u[3]*u[4]+u[2]
  BhpD Display : Display
  Gain : Gain  Gain=1000
  J - advance ratio : Fcn  Expr=u[1]/(u[2]*u[3])
  Mux : Mux
  Mux1 : Mux  Inputs=3
  Mux2 : Mux  Inputs=3
  Mux3 : Mux  Inputs=3
  Prop Eff : Display
  Prop Eff1 : Display
  Prop look up : Lookup_n-D  NumberOfTableDimensions=1  BreakpointsForDimension1=[0;0.048012249;0.060807878;0.079983697;0.105563205;0.133281193;0.157430152;0.178753263;0.199368443;0.215001671;0.227800237;0.245557257;0.273971426;0.300949171;0.327207235;0.352754431;0.371192944;0.390339388;0.409494645;0.433608354;0.457002383;0.472603298;0.491041811;0.509471512;0.534281402;0.552003172;0.576810125;0.598782418;0.619332973;0.645549913;0.671763915;0.690895672;0.717103799;0.745432781;0.760302266;0.778708467;0.799946391;0.819051711;0.845926644;0.867848999;0.888343743;0.903180915;0.92013013;0.934250559;0.947645432;0.961736487;0.970184657;0.980736057;0.986337817;0.992650444;0.994753675]  Table=[0;0.109900628;0.134509301;0.163123953;0.206809061;0.257361734;0.294163365;0.333794761;0.373442069;0.400753217;0.42674495;0.454008364;0.499012887;0.534367813;0.564206411;0.592677861;0.607477825;0.622261878;0.641195111;0.661400024;0.676088609;0.688186099;0.702986063;0.713636848;0.72829361;0.738960306;0.752234009;0.764188297;0.773408288;0.783884048;0.792976749;0.800845502;0.807172083;0.81206787;0.813116793;0.812703099;0.812225759;0.807646975;0.794594806;0.783037077;0.765978931;0.751814195;0.732069486;0.713771482;0.68719103;0.655062427;0.632742534;0.600693488;0.571521941;0.543717542;0.53398839]  InternalRulePriority=Speed  RndMeth=Simplest
  Shp : Fcn  Expr=0.95*u[1]
  Shp Display : Display
  Standard Temp : Fcn  Expr=59-0.00357*u[1]
  Standard Temp (F) : Display
  hp : Lookup_n-D  NumberOfTableDimensions=1  BreakpointsForDimension1=[12, 14, 16, 18, 20, 22, 24, 26, 28]  Table=[22.5, 19.3, 15.8, 12.8, 10.3, 7.8, 5.5, 3.25, 1.4]  InternalRulePriority=Speed  RndMeth=Simplest
  "hp' " : Display
  rpm to rps : Fcn  Expr=u[1]/60
  sdg : Display
  thrust to pounds : Fcn  Expr=u[3]*u[1]*550/(u[2])
  Out1 : Outport
  wires:
  hp/1 -> Gain/1
  Gain/1 -> [hp], Mux/3
  [ST] -> Standard Temp (F)/1
  Mux3/1 -> J - advance ratio/1
  [hp] -> "hp' "/1
  rpm to rps/1 -> Mux3/2
  Mux/1 -> BhpD/1
  Prop look up/1 -> [np], Prop Eff/1, Mux2/3
  J - advance ratio/1 -> Prop look up/1
  [np] -> Prop Eff1/1
  Shp/1 -> Shp Display/1, Mux2/1
  In1/1 -> hp/1, BhpB/1, BhpA/1
  In2/1 -> BhpA/2, BhpB/2, rpm to rps/1
  Mux1/1 -> Bhp/1
  BhpB/1 -> BhpB val/1, Mux/2
  Standard Temp/1 -> [ST], Mux1/2
  In3/1 -> Mux/4, Standard Temp/1
  thrust to pounds/1 -> Out1/1
  Bhp/1 -> Bhp Display/1, Shp/1
  In5/1 -> Mux2/2, Mux3/1
  Mux2/1 -> thrust to pounds/1
  BhpD/1 -> BhpD Display/1, Mux1/1
  BhpA/1 -> sdg/1, Mux/1
  In4/1 -> Mux1/3
  In6/1 -> Mux3/3

== system np/Subsystem24 ==
  note: This will give you hp'
  note: P=TV
      |
      | T = P/V (doesnt work with props)
      | T=Np*P/V (P, is shaft horse power or SHP)
  note: Ts=59F-0.00357*hp
  note: I think these are the vertical lines
  In1 : Inport
  In2 : Inport  Port=2
  In3 : Inport  Port=3
  In4 : Inport  Port=4
  In5 : Inport  Port=5
  In6 : Inport  Port=6
  Bhp : Fcn  Expr=u[1]*sqrt((460+u[2])/(460+u[3]))
  Bhp Display : Display
  BhpA : Lookup_n-D  BreakpointsForDimension1=[12;14;16;18;20;22;24;26;28]  BreakpointsForDimension2=[2000 2200 2400 2600 2700]  Table=[55 65 68 70 71;69 77 82 84 87;79 87 94 97 100;88 98 105 111 115;98 108 116 123 126;108 119 127 135 140;119 129 138 147 153;127 139 150 160 164;138 149 161 172 177]  InternalRulePriority=Speed  RndMeth=Simplest
      settings: InputPortMap=u0,u1
  BhpB : Lookup_n-D  BreakpointsForDimension1=[17 18 19 20 21 22 23 24 25 26 27 28 29]  BreakpointsForDimension2=[2000 2200 2400 2600 2700]  Table=[60 68 71 81 82;65 74 80 98 90;73 81 86 95 98;80 87 94 103 106;85 95 102 111 116;93 103 110 120 123;100 110 118 126 133;106 115 125 135 141;116 124 135 144 150;120 131 143 152 158;125 137 148 159 165;135 145 157 167 173;142 153 165 176 183]  InternalRulePriority=Speed  RndMeth=Simplest
      settings: InputPortMap=u0,u1
  BhpB val : Display
  BhpD : Fcn  Expr=(u[1]-u[2])/u[3]*u[4]+u[2]
  BhpD Display : Display
  Gain : Gain  Gain=1000
  J - advance ratio : Fcn  Expr=u[1]/(u[2]*u[3])
  Mux : Mux
  Mux1 : Mux  Inputs=3
  Mux2 : Mux  Inputs=3
  Mux3 : Mux  Inputs=3
  Prop Eff : Display
  Prop Eff1 : Display
  Prop look up : Lookup_n-D  NumberOfTableDimensions=1  BreakpointsForDimension1=[0;0.048012249;0.060807878;0.079983697;0.105563205;0.133281193;0.157430152;0.178753263;0.199368443;0.215001671;0.227800237;0.245557257;0.273971426;0.300949171;0.327207235;0.352754431;0.371192944;0.390339388;0.409494645;0.433608354;0.457002383;0.472603298;0.491041811;0.509471512;0.534281402;0.552003172;0.576810125;0.598782418;0.619332973;0.645549913;0.671763915;0.690895672;0.717103799;0.745432781;0.760302266;0.778708467;0.799946391;0.819051711;0.845926644;0.867848999;0.888343743;0.903180915;0.92013013;0.934250559;0.947645432;0.961736487;0.970184657;0.980736057;0.986337817;0.992650444;0.994753675]  Table=[0;0.109900628;0.134509301;0.163123953;0.206809061;0.257361734;0.294163365;0.333794761;0.373442069;0.400753217;0.42674495;0.454008364;0.499012887;0.534367813;0.564206411;0.592677861;0.607477825;0.622261878;0.641195111;0.661400024;0.676088609;0.688186099;0.702986063;0.713636848;0.72829361;0.738960306;0.752234009;0.764188297;0.773408288;0.783884048;0.792976749;0.800845502;0.807172083;0.81206787;0.813116793;0.812703099;0.812225759;0.807646975;0.794594806;0.783037077;0.765978931;0.751814195;0.732069486;0.713771482;0.68719103;0.655062427;0.632742534;0.600693488;0.571521941;0.543717542;0.53398839]  InternalRulePriority=Speed  RndMeth=Simplest
  Shp : Fcn  Expr=0.95*u[1]
  Shp Display : Display
  Standard Temp : Fcn  Expr=59-0.00357*u[1]
  Standard Temp (F) : Display
  hp : Lookup_n-D  NumberOfTableDimensions=1  BreakpointsForDimension1=[12, 14, 16, 18, 20, 22, 24, 26, 28]  Table=[22.5, 19.3, 15.8, 12.8, 10.3, 7.8, 5.5, 3.25, 1.4]  InternalRulePriority=Speed  RndMeth=Simplest
  "hp' " : Display
  rpm to rps : Fcn  Expr=u[1]/60
  sdg : Display
  thrust to pounds : Fcn  Expr=u[3]*u[1]*550/(u[2])
  Out1 : Outport
  wires:
  In6/1 -> Mux3/3
  In4/1 -> Mux1/3
  BhpA/1 -> Mux/1, sdg/1
  BhpD/1 -> Mux1/1, BhpD Display/1
  Mux2/1 -> thrust to pounds/1
  In5/1 -> Mux3/1, Mux2/2
  Bhp/1 -> Shp/1, Bhp Display/1
  thrust to pounds/1 -> Out1/1
  In3/1 -> Standard Temp/1, Mux/4
  Standard Temp/1 -> Mux1/2, [ST]
  BhpB/1 -> Mux/2, BhpB val/1
  Mux1/1 -> Bhp/1
  In2/1 -> rpm to rps/1, BhpB/2, BhpA/2
  In1/1 -> BhpA/1, BhpB/1, hp/1
  Shp/1 -> Mux2/1, Shp Display/1
  [np] -> Prop Eff1/1
  J - advance ratio/1 -> Prop look up/1
  Prop look up/1 -> Mux2/3, Prop Eff/1, [np]
  Mux/1 -> BhpD/1
  rpm to rps/1 -> Mux3/2
  [hp] -> "hp' "/1
  Mux3/1 -> J - advance ratio/1
  [ST] -> Standard Temp (F)/1
  Gain/1 -> Mux/3, [hp]
  hp/1 -> Gain/1

== system np/Subsystem25 ==
  note: I think these are the vertical lines
  note: Ts=59F-0.00357*hp
  note: P=TV
      |
      | T = P/V (doesnt work with props)
      | T=Np*P/V (P, is shaft horse power or SHP)
  note: This will give you hp'
  In1 : Inport
  In2 : Inport  Port=2
  In3 : Inport  Port=3
  In4 : Inport  Port=4
  In5 : Inport  Port=5
  In6 : Inport  Port=6
  Bhp : Fcn  Expr=u[1]*sqrt((460+u[2])/(460+u[3]))
  Bhp Display : Display
  BhpA : Lookup_n-D  BreakpointsForDimension1=[12;14;16;18;20;22;24;26;28]  BreakpointsForDimension2=[2000 2200 2400 2600 2700]  Table=[55 65 68 70 71;69 77 82 84 87;79 87 94 97 100;88 98 105 111 115;98 108 116 123 126;108 119 127 135 140;119 129 138 147 153;127 139 150 160 164;138 149 161 172 177]  InternalRulePriority=Speed  RndMeth=Simplest
      settings: InputPortMap=u0,u1
  BhpB : Lookup_n-D  BreakpointsForDimension1=[17 18 19 20 21 22 23 24 25 26 27 28 29]  BreakpointsForDimension2=[2000 2200 2400 2600 2700]  Table=[60 68 71 81 82;65 74 80 98 90;73 81 86 95 98;80 87 94 103 106;85 95 102 111 116;93 103 110 120 123;100 110 118 126 133;106 115 125 135 141;116 124 135 144 150;120 131 143 152 158;125 137 148 159 165;135 145 157 167 173;142 153 165 176 183]  InternalRulePriority=Speed  RndMeth=Simplest
      settings: InputPortMap=u0,u1
  BhpB val : Display
  BhpD : Fcn  Expr=(u[1]-u[2])/u[3]*u[4]+u[2]
  BhpD Display : Display
  Gain : Gain  Gain=1000
  J - advance ratio : Fcn  Expr=u[1]/(u[2]*u[3])
  Mux : Mux
  Mux1 : Mux  Inputs=3
  Mux2 : Mux  Inputs=3
  Mux3 : Mux  Inputs=3
  Prop Eff : Display
  Prop Eff1 : Display
  Prop look up : Lookup_n-D  NumberOfTableDimensions=1  BreakpointsForDimension1=[0;0.048012249;0.060807878;0.079983697;0.105563205;0.133281193;0.157430152;0.178753263;0.199368443;0.215001671;0.227800237;0.245557257;0.273971426;0.300949171;0.327207235;0.352754431;0.371192944;0.390339388;0.409494645;0.433608354;0.457002383;0.472603298;0.491041811;0.509471512;0.534281402;0.552003172;0.576810125;0.598782418;0.619332973;0.645549913;0.671763915;0.690895672;0.717103799;0.745432781;0.760302266;0.778708467;0.799946391;0.819051711;0.845926644;0.867848999;0.888343743;0.903180915;0.92013013;0.934250559;0.947645432;0.961736487;0.970184657;0.980736057;0.986337817;0.992650444;0.994753675]  Table=[0;0.109900628;0.134509301;0.163123953;0.206809061;0.257361734;0.294163365;0.333794761;0.373442069;0.400753217;0.42674495;0.454008364;0.499012887;0.534367813;0.564206411;0.592677861;0.607477825;0.622261878;0.641195111;0.661400024;0.676088609;0.688186099;0.702986063;0.713636848;0.72829361;0.738960306;0.752234009;0.764188297;0.773408288;0.783884048;0.792976749;0.800845502;0.807172083;0.81206787;0.813116793;0.812703099;0.812225759;0.807646975;0.794594806;0.783037077;0.765978931;0.751814195;0.732069486;0.713771482;0.68719103;0.655062427;0.632742534;0.600693488;0.571521941;0.543717542;0.53398839]  InternalRulePriority=Speed  RndMeth=Simplest
  Shp : Fcn  Expr=0.95*u[1]
  Shp Display : Display
  Standard Temp : Fcn  Expr=59-0.00357*u[1]
  Standard Temp (F) : Display
  hp : Lookup_n-D  NumberOfTableDimensions=1  BreakpointsForDimension1=[12, 14, 16, 18, 20, 22, 24, 26, 28]  Table=[22.5, 19.3, 15.8, 12.8, 10.3, 7.8, 5.5, 3.25, 1.4]  InternalRulePriority=Speed  RndMeth=Simplest
  "hp' " : Display
  rpm to rps : Fcn  Expr=u[1]/60
  sdg : Display
  thrust to pounds : Fcn  Expr=u[3]*u[1]*550/(u[2])
  Out1 : Outport
  wires:
  hp/1 -> Gain/1
  Gain/1 -> [hp], Mux/3
  [ST] -> Standard Temp (F)/1
  Mux3/1 -> J - advance ratio/1
  [hp] -> "hp' "/1
  rpm to rps/1 -> Mux3/2
  Mux/1 -> BhpD/1
  Prop look up/1 -> [np], Prop Eff/1, Mux2/3
  J - advance ratio/1 -> Prop look up/1
  [np] -> Prop Eff1/1
  Shp/1 -> Shp Display/1, Mux2/1
  In1/1 -> hp/1, BhpB/1, BhpA/1
  In2/1 -> BhpA/2, BhpB/2, rpm to rps/1
  Mux1/1 -> Bhp/1
  BhpB/1 -> BhpB val/1, Mux/2
  Standard Temp/1 -> [ST], Mux1/2
  In3/1 -> Mux/4, Standard Temp/1
  thrust to pounds/1 -> Out1/1
  Bhp/1 -> Bhp Display/1, Shp/1
  In5/1 -> Mux2/2, Mux3/1
  Mux2/1 -> thrust to pounds/1
  BhpD/1 -> BhpD Display/1, Mux1/1
  BhpA/1 -> sdg/1, Mux/1
  In4/1 -> Mux1/3
  In6/1 -> Mux3/3
